simulink model "rlCartPole"  (R2021b)
settings: Solver=VariableStepAuto  StartTime=0.0  StopTime=Tf  RelTol=1e-3
PreLoadFcn:
  | qubeInit
values from neighbouring files (symbols this model uses):
  g = 9.81    [qubeInit.m]
  Jm = 4e-6    (= 4e-06)    [qubeInit.m]
  Klqr = lqr(A,B,Q,R)    [qubeInit.m]
  Lp = 0.129    [qubeInit.m]
  Lr = 0.085    [qubeInit.m]
  maxLimit = 10    [qubeInit.m]
  Mh = 0.0106    [qubeInit.m]
  minLimit = -10    [qubeInit.m]
  Mp = 0.024    [qubeInit.m]
  Mr = 0.095    [qubeInit.m]
  Rh = 0.0111    [qubeInit.m]
  stepFreq = 1    [qubeInit.m]
  stepSize = 0    [qubeInit.m]
  thetaMax = 135    [qubeInit.m]
  Ts = 0.02    [qubeInit.m]
undefined symbols (not defined in the file or in its folder): X, Y, Z
libraries: sm_lib x16, nesl_utility x8, fl_lib x4, rllib x1, ee_lib x1, simulink x1
settings Model: Creator=ndoshi  LastModifiedBy=hooverrj
settings SolverCC: AlgebraicLoopSolver=TrustRegion
settings DataIOCC: TimeSaveName=T  SignalLoggingName=LoggedSigs
settings DebuggingCC: SFMachineParentedDataDiag=warning  ArithmeticOperatorsInVariantConditions=warning
settings SFSimCC: CustomCodeUndefinedFunction=UseInterfaceOnly
settings ExplorerConfigSet: InternalSimMechanicsExplorerSettings="<ExplorerConfiguration><canonicalview>default</canonicalview><AnimationSetting><BasePlaybackSpeed>1.0</BasePlaybackSpeed><PlaybackSpeedFactor>1.0</PlaybackSpeedFactor></AnimationSetting><TilePanel><TileInfo><Tiles Columns=\"1\" Count=\"1\" Rows=\"1\"><Column Weight=\"1\"/><Row Weight=\"1\"/><Tile Height=\"1\" Width=\"1\" X=\"0\" Y=\"0\"/></Tiles></TileInfo><SceneInfo><SceneViewer><BGColor><R>0.60000002384185791</R><G>0.60000002384185791</G><B>0.60000002384185791</B></BGColor><Camera><DoPerspective>on</DoPerspective><Position><X>0.431019807204840122</X><Y>-0.00147907084386321701</Y><Z>0.0248156253974509827</Z></Position><Center><X>0.234686259791210938</X><Y>-0.00147907084386321701</Y><Z>0.0248156253974509827</Z></Center><Up><X>-0</X><Y>0</Y><Z>1</Z></Up><ViewLimDist>1</ViewLimDist><YLim>0.466307658154998583</YLim><XLim>0.677990771454933028</XLim></Camera></SceneViewer></SceneInfo></TilePanel><MechEditorPanel><Cameras><Camera><Id>Camera1</Id><Value><Name>Camera1</Name><NativeCamera><PositionTrackingFeature>Environment.Plant.World_Frame.W</PositionTrackingFeature><CenterTrackingFeature>Environment.Plant.World_Frame.W</CenterTrackingFeature><UpVectorTrackingFeature>Environment.Plant.World_Frame.W</UpVectorTrackingFeature><CenterTrackingOrigin>on</CenterTrackingOrigin><UpVectorTrackingDirection>+X</UpVectorTrackingDirection></NativeCamera></Value></Camera></Cameras><GfxPanelCameraMap><MapElement CameraMLId=\"Camera1\" GfxPanelIndex=\"0\"/></GfxPanelCameraMap><VideoCreator><PlaybackSpeedRatio>1.0</PlaybackSpeedRatio><FrameRate>30</FrameRate><VideoFormat>Motion JPEG AVI</VideoFormat><FrameSize>auto</FrameSize></VideoCreator></MechEditorPanel></ExplorerConfiguration>"

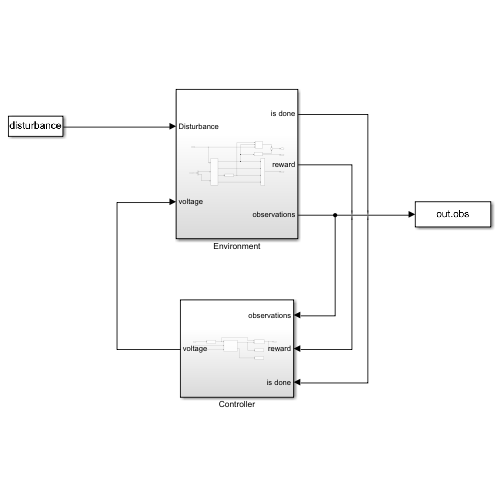
[thumbnail: Simulink's stored preview of the top-level diagram]
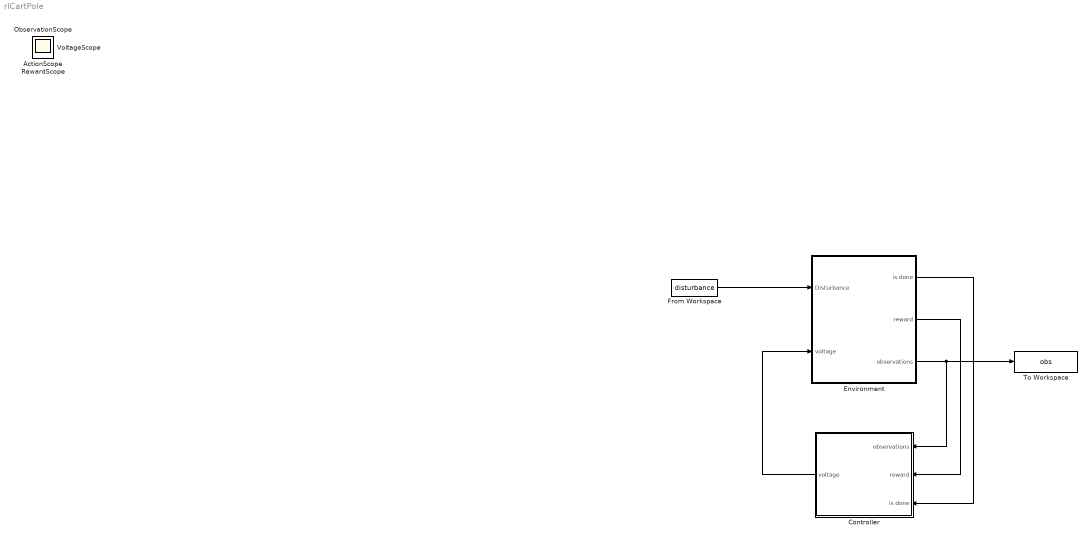
== system rlCartPole ==
  Controller : Subsystem
  Environment : Subsystem
  From Workspace : FromWorkspace  VariableName=disturbance
  To Workspace : ToWorkspace  VariableName=obs  SaveFormat=Timeseries  SampleTime=-1
  ActionScope : Scope
  ObservationScope : Scope
  RewardScope : Scope
  VoltageScope : Scope
  wires:
  Environment/3(observations) -> Controller/1(observations), To Workspace/1
  Environment/2(reward) -> Controller/2(reward)
  Environment/1(is done) -> Controller/3(is done)
  Controller/1(voltage) -> Environment/2(voltage)
  From Workspace/1 -> Environment/1(Disturbance)

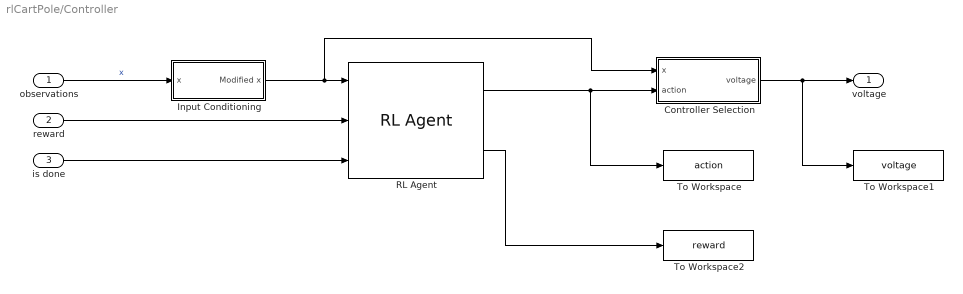
== system rlCartPole/Controller ==
  observations : Inport
  reward : Inport  Port=2
  is done : Inport  Port=3
  Controller Selection : Subsystem  Variant=on
  Input Conditioning : Subsystem
  RL Agent : rllib/RL Agent  Agent=agent  ExternalActionAsInput=off  ProvideCumRwd=on  TreatAsDirectFeedthrough=on
  To Workspace : ToWorkspace  VariableName=action  SaveFormat=Timeseries  SampleTime=-1
  To Workspace1 : ToWorkspace  VariableName=voltage  SaveFormat=Timeseries  SampleTime=-1
  To Workspace2 : ToWorkspace  VariableName=reward  SaveFormat=Timeseries  SampleTime=-1
  voltage : Outport
  wires:
  reward/1 -> RL Agent/2
  is done/1 -> RL Agent/3
  Controller Selection/1(voltage) -> To Workspace1/1, voltage/1
  RL Agent/1 -> To Workspace/1, Controller Selection/2(action)
  Input Conditioning/1(Modified x) -> Controller Selection/1(x), RL Agent/1
  observations/1 -> Input Conditioning/1(x)  "x"
  RL Agent/2 -> To Workspace2/1

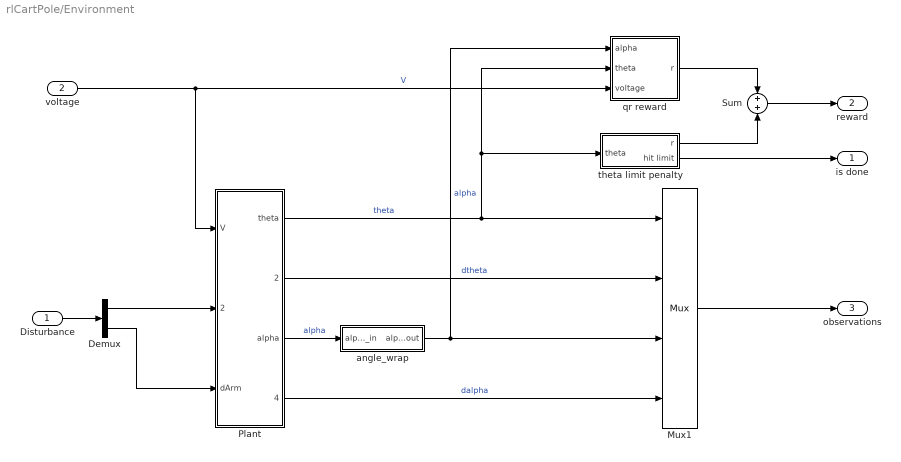
== system rlCartPole/Environment ==
  Disturbance : Inport
  voltage : Inport  Port=2
  Demux : Demux  Outputs=2
  Mux1 : Mux
  Plant : Subsystem
  Sum : Sum
  angle_wrap : Subsystem
  qr reward : Subsystem
  theta limit penalty : Subsystem
  is done : Outport  VectorParamsAs1DForOutWhenUnconnected=off
  reward : Outport  Port=2  VectorParamsAs1DForOutWhenUnconnected=off
  observations : Outport  Port=3  VectorParamsAs1DForOutWhenUnconnected=off
  wires:
  Mux1/1 -> observations/1
  Plant/4(alpha_dot) -> Mux1/4  "dalpha"
  Plant/3(alpha) -> angle_wrap/1(alpha_in)  "alpha"
  Plant/1(theta) -> Mux1/1, qr reward/2(theta), theta limit penalty/1(theta)  "theta"
  angle_wrap/1(alpha_out) -> Mux1/3, qr reward/1(alpha)  "alpha"
  Plant/2(theta_dot) -> Mux1/2  "dtheta"
  Sum/1 -> reward/1
  theta limit penalty/2(hit limit) -> is done/1
  voltage/1 -> Plant/1(V), qr reward/3(voltage)  "V"
  qr reward/1(r) -> Sum/1
  theta limit penalty/1(r) -> Sum/2
  Demux/2 -> Plant/3(dArm)
  Demux/1 -> Plant/2(dPend)
  Disturbance/1 -> Demux/1

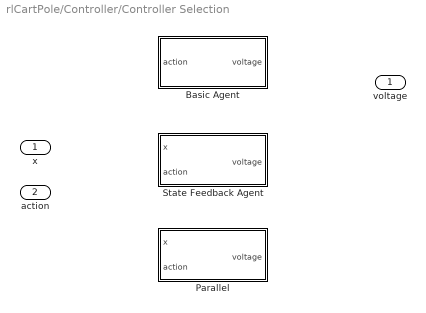
== system rlCartPole/Controller/Controller Selection ==
  x : Inport
  action : Inport  Port=2
  Basic Agent : Subsystem  VariantControl=VSS_CONTROL_BASIC
  Parallel : Subsystem  VariantControl=VSS_CONTROL_FF
  State Feedback Agent : Subsystem  VariantControl=VSS_CONTROL_STATE
  voltage : Outport

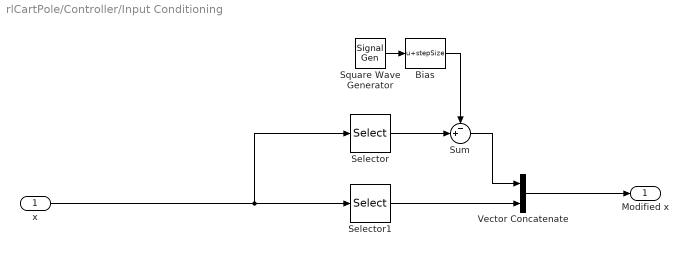
== system rlCartPole/Controller/Input Conditioning ==
  x : Inport
  Bias : Bias  Bias=stepSize
  Selector : Selector  InputPortWidth=4  IndexOptions=Index vector (dialog)  Indices=1  OutputSizes=1
  Selector1 : Selector  InputPortWidth=4  IndexOptions=Index vector (dialog)  Indices=[2 3 4]  OutputSizes=1
  Square Wave Generator : SignalGenerator  WaveForm=square  Amplitude=stepSize  Frequency=stepFreq
  Sum : Sum  Inputs=-+|
  Vector Concatenate : Concatenate
  Modified x : Outport
  wires:
  Vector Concatenate/1 -> Modified x/1
  x/1 -> Selector1/1, Selector/1
  Square Wave Generator/1 -> Bias/1
  Sum/1 -> Vector Concatenate/1
  Selector1/1 -> Vector Concatenate/2
  Selector/1 -> Sum/2
  Bias/1 -> Sum/1

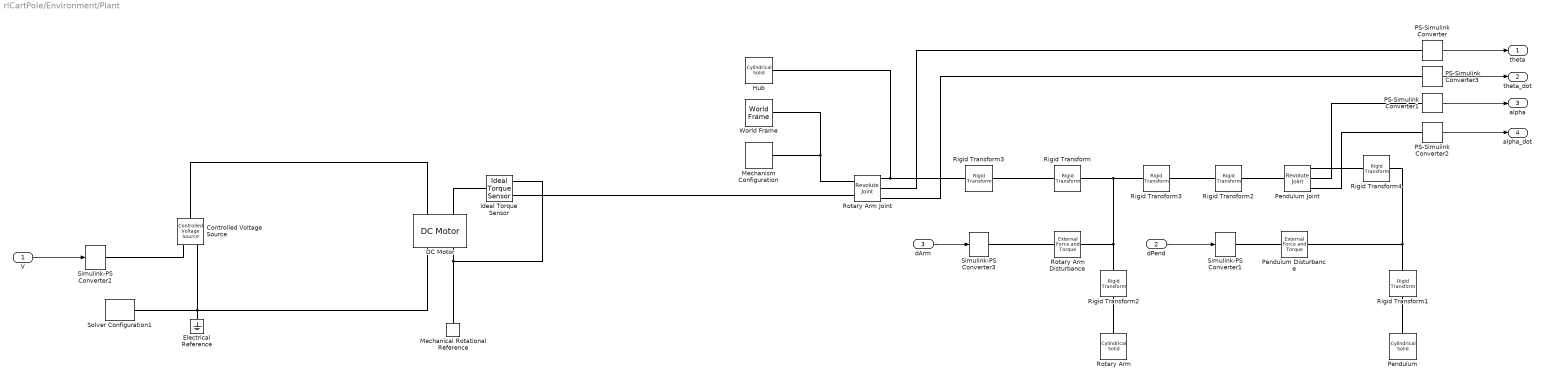
== system rlCartPole/Environment/Plant ==
  V : Inport
  dPend : Inport  Port=2
  dArm : Inport  Port=3
  Controlled Voltage Source : fl_lib/Electrical/Electrical Sources/Controlled Voltage Source
  DC Motor : ee_lib/Electromechanical/Brushed Motors/DC Motor  field_option=ee.enum.field_option.pm  Rf=100 Ohm  Lf=1 H  Laf=0.15 H  If0=0 A  parameterization=1  Ra=Rm Ohm  La=Lm mH  emf_or_torque=1  Kv=Km V/(rad/s)  Ki=6.876e-4 N*m/A  T_stall=0.24e-3 N*m  w_max=19100 rpm  w_rated=15000 rpm  P_rated=0.08 W  V_rated=1.5 V  lam_param=1  i_noload=0 A  V_i_noload=1.5 V  J=Jm kg*m^2  lam=0 N*m/(rad/s)  speed0=0 rpm  enable_fault_armature=simscape.enum.onoff.off  rev_faulted=1 / 3  G_faulted_armature=1e-5 S  fault_trigger_armature=ee.enum.faults.faultTrigger.temporal  t_fault_armature=1 s  max_permissible_current_armature=inf A  t_fail_on_current_armature=1 s  enable_fault_field=simscape.enum.onoff.off  G_faulted_field=1e-5 S  fault_trigger_field=ee.enum.faults.faultTrigger.temporal  t_fault_field=1 s  max_permissible_current_field=inf A  t_fail_on_current_field=1 s  fault_action=simscape.enum.assert.action.none  alpha=3.93e-3 1/K  Tmeas=25 degC  thermal_mass=100 J/K  initial_temperature=25 degC
  Electrical Reference : fl_lib/Electrical/Electrical Elements/Electrical Reference
  Hub : sm_lib/Body Elements/Cylindrical Solid  GraphicAmbientColor=[0.15 0.15 0.15 1.0]  BasedOnType=Mass  CenterOfMass=[0 0 0]  CenterOfMassUnits=m  GraphicDiffuseColor=[0.5 0.5 0.5]  CylinderLength=Rh/2  CylinderLengthUnits=m  CylinderRadius=Rh  CylinderRadiusUnits=m  Density=1000  DensityUnits=kg/m^3  DoExposeReferenceFrame=on  GraphicEmissiveColor=[0.0 0.0 0.0 1.0]  ExportEntireGeometry=off  SerializedFrames=<Frames/>  MarkerShape=Sphere  MarkerSize=10  GraphicType=FromGeometry  InertiaType=CalculateFromGeometry  Mass=Mh  MassUnits=kg  MomentsOfInertia=[1 1 1]  MomentsOfInertiaUnits=kg*m^2  GraphicOpacity=1.0  ProductsOfInertia=[0 0 0]  ProductsOfInertiaUnits=kg*m^2  GraphicShininess=75  GraphicSpecularColor=[0.5 0.5 0.5 1.0]  GraphicVisPropType=SimpleVisualProperties
  Ideal Torque Sensor : fl_lib/Mechanical/Mechanical Sensors/Ideal Torque Sensor
  Mechanical Rotational Reference : fl_lib/Mechanical/Rotational Elements/Mechanical Rotational Reference
  Mechanism Configuration : sm_lib/Utilities/Mechanism Configuration  UniformGravity=Constant  GravityVector=[0 0 -g]  GravityUnits=m/s^2  LinearizationDelta=0.001  JointModeTransitionNonlinearIterations=2
  PS-Simulink Converter{,1..3} (4 alike) : nesl_utility/PS-Simulink Converter  PhysicalDomain=network_engine_domain  SubClassName=ps_output  LeftPortType=input  RightPortType=output  PseudoPeriodic=off  Frequencies=[]  Unit=1  AffineConversion=off
      settings: SourceProductBaseCode=PW,SS
  Pendulum : sm_lib/Body Elements/Cylindrical Solid  GraphicAmbientColor=[0.15 0.15 0.15 1.0]  BasedOnType=Mass  CenterOfMass=[0 0 0]  CenterOfMassUnits=m  GraphicDiffuseColor=[0.8 0.0 0.2]  CylinderLength=Lp  CylinderLengthUnits=m  CylinderRadius=0.005  CylinderRadiusUnits=m  Density=1000  DensityUnits=kg/m^3  DoExposeReferenceFrame=on  GraphicEmissiveColor=[0.0 0.0 0.0 1.0]  ExportEntireGeometry=off  SerializedFrames=<Frames/>  MarkerShape=Sphere  MarkerSize=10  GraphicType=FromGeometry  InertiaType=CalculateFromGeometry  Mass=Mp  MassUnits=kg  MomentsOfInertia=[1 1 1]  MomentsOfInertiaUnits=kg*m^2  GraphicOpacity=1.0  ProductsOfInertia=[0 0 0]  ProductsOfInertiaUnits=kg*m^2  GraphicShininess=75  GraphicSpecularColor=[0.5 0.5 0.5 1.0]  GraphicVisPropType=SimpleVisualProperties
  Pendulum Disturbance : sm_lib/Forces and Torques/External Force and Torque  ForceResolutionFrame=AttachedFrame  EnableForceX=off  EnableForceY=on  EnableForceZ=off  EnableForce=off  TorqueResolutionFrame=AttachedFrame  EnableTorqueX=off  EnableTorqueY=off  EnableTorqueZ=off  EnableTorque=off
  Pendulum Joint : sm_lib/Joints/Revolute Joint  JointMode=Normal  SenseConstraintForce=off  SenseConstraintForceX=off  SenseConstraintForceY=off  SenseConstraintForceZ=off  SenseConstraintTorque=off  SenseConstraintTorqueX=off  SenseConstraintTorqueY=off  SenseConstraintTorqueZ=off  SenseTotalForce=off  SenseTotalForceX=off  SenseTotalForceY=off  SenseTotalForceZ=off  SenseTotalTorque=off  SenseTotalTorqueX=off  SenseTotalTorqueY=off  SenseTotalTorqueZ=off  CompositeWrenchDir=FollowerOnBase  CompositeWrenchFrame=BaseFrame  EquilibriumPosition=0  EquilibriumPositionUnits=deg  SpringStiffness=0  SpringStiffnessUnits=N*m/deg  DampingCoefficient=Dp  DampingCoefficientUnits=N*m/(rad/s)  TorqueActuationMode=NoTorque  MotionActuationMode=ComputedMotion  SensePosition=on  SenseVelocity=on  SenseAcceleration=off  SenseTorqueForce=off  SenseLowerLimitTorqueForce=off  SenseUpperLimitTorqueForce=off  LowerLimitSpecify=off  LowerLimitBound=-90  LowerLimitBoundUnits=deg  LowerLimitStiffness=1e4  LowerLimitStiffnessUnits=N*m/deg  LowerLimitDamping=10  LowerLimitDampingUnits=N*m/(deg/s)  LowerLimitTransitionRegionWidth=0.1  LowerLimitTransitionRegionWidthUnits=deg  UpperLimitSpecify=off  UpperLimitBound=90  UpperLimitBoundUnits=deg  UpperLimitStiffness=1e4  UpperLimitStiffnessUnits=N*m/deg  UpperLimitDamping=10  UpperLimitDampingUnits=N*m/(deg/s)  UpperLimitTransitionRegionWidth=0.1  UpperLimitTransitionRegionWidthUnits=deg  PositionTargetSpecify=on  PositionTargetPriority=High  PositionTargetValue=alpha0  PositionTargetValueUnits=deg  VelocityTargetSpecify=off  VelocityTargetPriority=High  VelocityTargetValue=0  VelocityTargetValueUnits=deg/s
  Rigid Transform : sm_lib/Frames and Transforms/Rigid Transform  TranslationMethod=StandardAxis  TranslationStandardOffset=Lr/2  TranslationLengthUnit=m  TranslationStandardAxis=-X  TranslationCartesianOffset=[0 0 0]  TranslationROffset=0  TranslationROffsetUnits=m  TranslationZOffset=0  TranslationZOffsetUnits=m  TranslationThetaOffset=0  TranslationThetaOffsetUnits=deg  RotationMethod=None  RotationAngleUnits=deg  RotationStandardAxis=+Z  RotationAngle=0.0  RotationArbitraryAxis=[0 0 1]  FollAlignAxisA=+X  BaseAlignAxisA=+Y  FollAlignAxisB=+Y  BaseAlignAxisB=+Z  RotationSequenceAxes=FollowerAxes  RotationSequence=XYX  RotationSequenceAngles=[0 0 0]  RotationSequenceAnglesUnits=deg  RotationMatrix=[1 0 0; 0 1 0; 0 0 1]
  Rigid Transform1 : sm_lib/Frames and Transforms/Rigid Transform  TranslationMethod=None  TranslationStandardOffset=0  TranslationLengthUnit=m  TranslationStandardAxis=+Z  TranslationCartesianOffset=[0 0 0]  TranslationROffset=0  TranslationROffsetUnits=m  TranslationZOffset=0  TranslationZOffsetUnits=m  TranslationThetaOffset=0  TranslationThetaOffsetUnits=deg  RotationMethod=StandardAxis  RotationAngleUnits=deg  RotationStandardAxis=-Y  RotationAngle=90  RotationArbitraryAxis=[0 0 1]  FollAlignAxisA=+X  BaseAlignAxisA=+Y  FollAlignAxisB=+Y  BaseAlignAxisB=+Z  RotationSequenceAxes=FollowerAxes  RotationSequence=XYX  RotationSequenceAngles=[0 0 0]  RotationSequenceAnglesUnits=deg  RotationMatrix=[1 0 0; 0 1 0; 0 0 1]
  Rigid Transform2 : sm_lib/Frames and Transforms/Rigid Transform  TranslationMethod=None  TranslationStandardOffset=0  TranslationLengthUnit=m  TranslationStandardAxis=+Z  TranslationCartesianOffset=[0 0 0]  TranslationROffset=0  TranslationROffsetUnits=m  TranslationZOffset=0  TranslationZOffsetUnits=m  TranslationThetaOffset=0  TranslationThetaOffsetUnits=deg  RotationMethod=StandardAxis  RotationAngleUnits=deg  RotationStandardAxis=-Y  RotationAngle=90  RotationArbitraryAxis=[0 0 1]  FollAlignAxisA=+X  BaseAlignAxisA=+Y  FollAlignAxisB=+Y  BaseAlignAxisB=+Z  RotationSequenceAxes=FollowerAxes  RotationSequence=XYX  RotationSequenceAngles=[0 0 0]  RotationSequenceAnglesUnits=deg  RotationMatrix=[1 0 0; 0 1 0; 0 0 1]
  Rigid Transform3 : sm_lib/Frames and Transforms/Rigid Transform  TranslationMethod=StandardAxis  TranslationStandardOffset=Rh/2  TranslationLengthUnit=m  TranslationStandardAxis=-Z  TranslationCartesianOffset=[0 0 0]  TranslationROffset=0  TranslationROffsetUnits=m  TranslationZOffset=0  TranslationZOffsetUnits=m  TranslationThetaOffset=0  TranslationThetaOffsetUnits=deg  RotationMethod=None  RotationAngleUnits=deg  RotationStandardAxis=+Z  RotationAngle=0.0  RotationArbitraryAxis=[0 0 1]  FollAlignAxisA=+X  BaseAlignAxisA=+Y  FollAlignAxisB=+Y  BaseAlignAxisB=+Z  RotationSequenceAxes=FollowerAxes  RotationSequence=XYX  RotationSequenceAngles=[0 0 0]  RotationSequenceAnglesUnits=deg  RotationMatrix=[1 0 0; 0 1 0; 0 0 1]
  Rigid Transform2 : sm_lib/Frames and Transforms/Rigid Transform  TranslationMethod=StandardAxis  TranslationStandardOffset=Lr/2  TranslationLengthUnit=m  TranslationStandardAxis=+Z  TranslationCartesianOffset=[0 0 0]  TranslationROffset=0  TranslationROffsetUnits=m  TranslationZOffset=0  TranslationZOffsetUnits=m  TranslationThetaOffset=0  TranslationThetaOffsetUnits=deg  RotationMethod=None  RotationAngleUnits=deg  RotationStandardAxis=-X  RotationAngle=90  RotationArbitraryAxis=[0 0 1]  FollAlignAxisA=+X  BaseAlignAxisA=+Y  FollAlignAxisB=+Y  BaseAlignAxisB=+Z  RotationSequenceAxes=FollowerAxes  RotationSequence=XYX  RotationSequenceAngles=[0 0 0]  RotationSequenceAnglesUnits=deg  RotationMatrix=[1 0 0; 0 1 0; 0 0 1]
  Rigid Transform3 : sm_lib/Frames and Transforms/Rigid Transform  TranslationMethod=None  TranslationStandardOffset=0  TranslationLengthUnit=m  TranslationStandardAxis=+Z  TranslationCartesianOffset=[0 0 0]  TranslationROffset=0  TranslationROffsetUnits=m  TranslationZOffset=0  TranslationZOffsetUnits=m  TranslationThetaOffset=0  TranslationThetaOffsetUnits=deg  RotationMethod=StandardAxis  RotationAngleUnits=deg  RotationStandardAxis=+Y  RotationAngle=90  RotationArbitraryAxis=[0 0 1]  FollAlignAxisA=+X  BaseAlignAxisA=+Y  FollAlignAxisB=+Y  BaseAlignAxisB=+Z  RotationSequenceAxes=FollowerAxes  RotationSequence=XYX  RotationSequenceAngles=[0 0 0]  RotationSequenceAnglesUnits=deg  RotationMatrix=[1 0 0; 0 1 0; 0 0 1]
  Rigid Transform4 : sm_lib/Frames and Transforms/Rigid Transform  TranslationMethod=StandardAxis  TranslationStandardOffset=Lp/2  TranslationLengthUnit=m  TranslationStandardAxis=-X  TranslationCartesianOffset=[0 0 0]  TranslationROffset=0  TranslationROffsetUnits=m  TranslationZOffset=0  TranslationZOffsetUnits=m  TranslationThetaOffset=0  TranslationThetaOffsetUnits=deg  RotationMethod=None  RotationAngleUnits=deg  RotationStandardAxis=+X  RotationAngle=90  RotationArbitraryAxis=[0 0 1]  FollAlignAxisA=+X  BaseAlignAxisA=+Y  FollAlignAxisB=+Y  BaseAlignAxisB=+Z  RotationSequenceAxes=FollowerAxes  RotationSequence=XYX  RotationSequenceAngles=[0 0 0]  RotationSequenceAnglesUnits=deg  RotationMatrix=[1 0 0; 0 1 0; 0 0 1]
  Rotary Arm : sm_lib/Body Elements/Cylindrical Solid  GraphicAmbientColor=[0.15 0.15 0.15 1.0]  BasedOnType=Mass  CenterOfMass=[0 0 0]  CenterOfMassUnits=m  GraphicDiffuseColor=[0.5 0.5 0.5]  CylinderLength=Lr  CylinderLengthUnits=m  CylinderRadius=0.003  CylinderRadiusUnits=m  Density=1000  DensityUnits=kg/m^3  DoExposeReferenceFrame=on  GraphicEmissiveColor=[0.0 0.0 0.0 1.0]  ExportEntireGeometry=off  SerializedFrames=<Frames/>  MarkerShape=Sphere  MarkerSize=10  GraphicType=FromGeometry  InertiaType=CalculateFromGeometry  Mass=Mr  MassUnits=kg  MomentsOfInertia=[1 1 1]  MomentsOfInertiaUnits=kg*m^2  GraphicOpacity=1.0  ProductsOfInertia=[0 0 0]  ProductsOfInertiaUnits=kg*m^2  GraphicShininess=75  GraphicSpecularColor=[0.5 0.5 0.5 1.0]  GraphicVisPropType=SimpleVisualProperties
  Rotary Arm Disturbance : sm_lib/Forces and Torques/External Force and Torque  ForceResolutionFrame=AttachedFrame  EnableForceX=off  EnableForceY=on  EnableForceZ=off  EnableForce=off  TorqueResolutionFrame=AttachedFrame  EnableTorqueX=off  EnableTorqueY=off  EnableTorqueZ=off  EnableTorque=off
  Rotary Arm Joint : sm_lib/Joints/Revolute Joint  JointMode=Normal  SenseConstraintForce=off  SenseConstraintForceX=off  SenseConstraintForceY=off  SenseConstraintForceZ=off  SenseConstraintTorque=off  SenseConstraintTorqueX=off  SenseConstraintTorqueY=off  SenseConstraintTorqueZ=off  SenseTotalForce=off  SenseTotalForceX=off  SenseTotalForceY=off  SenseTotalForceZ=off  SenseTotalTorque=off  SenseTotalTorqueX=off  SenseTotalTorqueY=off  SenseTotalTorqueZ=off  CompositeWrenchDir=FollowerOnBase  CompositeWrenchFrame=BaseFrame  EquilibriumPosition=0  EquilibriumPositionUnits=deg  SpringStiffness=0  SpringStiffnessUnits=N*m/deg  DampingCoefficient=Dr  DampingCoefficientUnits=N*m/(rad/s)  TorqueActuationMode=InputTorque  MotionActuationMode=ComputedMotion  SensePosition=on  SenseVelocity=on  SenseAcceleration=off  SenseTorqueForce=off  SenseLowerLimitTorqueForce=off  SenseUpperLimitTorqueForce=off  LowerLimitSpecify=off  LowerLimitBound=-90  LowerLimitBoundUnits=deg  LowerLimitStiffness=1e4  LowerLimitStiffnessUnits=N*m/deg  LowerLimitDamping=10  LowerLimitDampingUnits=N*m/(deg/s)  LowerLimitTransitionRegionWidth=0.1  LowerLimitTransitionRegionWidthUnits=deg  UpperLimitSpecify=off  UpperLimitBound=90  UpperLimitBoundUnits=deg  UpperLimitStiffness=1e4  UpperLimitStiffnessUnits=N*m/deg  UpperLimitDamping=10  UpperLimitDampingUnits=N*m/(deg/s)  UpperLimitTransitionRegionWidth=0.1  UpperLimitTransitionRegionWidthUnits=deg  PositionTargetSpecify=on  PositionTargetPriority=High  PositionTargetValue=theta0  PositionTargetValueUnits=deg  VelocityTargetSpecify=off  VelocityTargetPriority=High  VelocityTargetValue=0  VelocityTargetValueUnits=deg/s
  Simulink-PS Converter1 : nesl_utility/Simulink-PS Converter  PhysicalDomain=network_engine_domain  SubClassName=ps_input  LeftPortType=input  RightPortType=output  PseudoPeriodic=off  Frequencies=[]  NoiseDistribution=none  NoiseParameters=[]  Unit=1  AffineConversion=off  FilteringAndDerivatives=zero  SimscapeFilterOrder=1  InputFilterTimeConstant=0.001  UdotUserProvided=1
      settings: SourceProductBaseCode=PW,SS
  Simulink-PS Converter2 : nesl_utility/Simulink-PS Converter  PhysicalDomain=network_engine_domain  SubClassName=ps_input  LeftPortType=input  RightPortType=output  PseudoPeriodic=off  Frequencies=[]  NoiseDistribution=none  NoiseParameters=[]  Unit=1  AffineConversion=off  FilteringAndDerivatives=zero  SimscapeFilterOrder=1  InputFilterTimeConstant=0.001  UdotUserProvided=1
      settings: SourceProductBaseCode=PW,SS
  Simulink-PS Converter3 : nesl_utility/Simulink-PS Converter  PhysicalDomain=network_engine_domain  SubClassName=ps_input  LeftPortType=input  RightPortType=output  PseudoPeriodic=off  Frequencies=[]  NoiseDistribution=none  NoiseParameters=[]  Unit=1  AffineConversion=off  FilteringAndDerivatives=zero  SimscapeFilterOrder=1  InputFilterTimeConstant=0.001  UdotUserProvided=1
      settings: SourceProductBaseCode=PW,SS
  Solver Configuration1 : nesl_utility/Solver Configuration  PhysicalDomain=network_engine_domain  SubClassName=solver  LeftPortType=input  RightPortType=generic  Tones=[]  Harmonics=[]  SimulateNoise=off  Profile=off  UseLocalSampling=off  EnableSwitchedLinearOptims=on  FrequencyDomain=off  UseCCode=off  RelTol=0.001  AbsTol=1e-06  MinStep=1e-09  ToWorkspace=off  RevertToSquareIcSolve=off  NumHomotopyIterations=100  PhasorMode=off  PhasorModeNumHarmonics=1  DoDC=off  ResidualTolerance=1e-09  UseLocalSolver=off  LocalSolverChoice=NE_BACKWARD_EULER_ADVANCER  LocalSolverSampleTime=0.001  DoFixedCost=off  MaxNonlinIter=3  MaxModeIter=2  ComputeImpulses=off  ImpulseIterations=2  LinearAlgebra=Sparse  EquationFormulation=NE_TIME_EF  DelaysMemoryBudget=1024  AutomaticFiltering=on  FilteringTimeConstant=0.001  PartitionStorageMethod=AS_NEEDED  PartitionMemoryBudget=1024  PartitionMethod=FAST
      settings: SourceProductBaseCode=PW,SS
  World Frame : sm_lib/Frames and Transforms/World Frame
  theta : Outport  VectorParamsAs1DForOutWhenUnconnected=off
  theta_dot : Outport  Port=2  VectorParamsAs1DForOutWhenUnconnected=off
  alpha : Outport  Port=3  VectorParamsAs1DForOutWhenUnconnected=off
  alpha_dot : Outport  Port=4  VectorParamsAs1DForOutWhenUnconnected=off
  wires:
  PS-Simulink Converter1/1 -> alpha/1
  PS-Simulink Converter/1 -> theta/1
  dPend/1 -> Simulink-PS Converter1/1
  PS-Simulink Converter2/1 -> alpha_dot/1
  PS-Simulink Converter3/1 -> theta_dot/1
  V/1 -> Simulink-PS Converter2/1
  dArm/1 -> Simulink-PS Converter3/1
  connections:
  Rotary Arm Disturbance/RConn1 -- Rigid Transform2/RConn1 -- Rigid Transform/LConn1 -- Rigid Transform3/LConn1
  World Frame/RConn1 -- Rotary Arm Joint/LConn1 -- Mechanism Configuration/RConn1
  Pendulum Joint/RConn1 -- Rigid Transform4/LConn1
  Rigid Transform4/RConn1 -- Rigid Transform1/RConn1 -- Pendulum Disturbance/RConn1
  Pendulum Joint/RConn2 -- PS-Simulink Converter1/LConn1
  PS-Simulink Converter/LConn1 -- Rotary Arm Joint/RConn2
  Simulink-PS Converter1/RConn1 -- Pendulum Disturbance/LConn1
  Pendulum Joint/RConn3 -- PS-Simulink Converter2/LConn1
  PS-Simulink Converter3/LConn1 -- Rotary Arm Joint/RConn3
  Rigid Transform2/RConn1 -- Pendulum Joint/LConn1
  Rigid Transform3/RConn1 -- Rigid Transform2/LConn1
  Simulink-PS Converter3/RConn1 -- Rotary Arm Disturbance/LConn1
  Simulink-PS Converter2/RConn1 -- Controlled Voltage Source/RConn1
  Ideal Torque Sensor/LConn1 -- DC Motor/LConn2
  DC Motor/RConn2 -- Ideal Torque Sensor/RConn1 -- Mechanical Rotational Reference/LConn1
  Controlled Voltage Source/LConn1 -- DC Motor/LConn1
  DC Motor/RConn1 -- Electrical Reference/LConn1 -- Solver Configuration1/RConn1 -- Controlled Voltage Source/RConn2
  Rigid Transform1/LConn1 -- Pendulum/RConn1
  Rigid Transform2/LConn1 -- Rotary Arm/RConn1
  Hub/RConn1 -- Rigid Transform3/RConn1 -- Rotary Arm Joint/RConn1
  Rigid Transform/RConn1 -- Rigid Transform3/LConn1
  Rotary Arm Joint/LConn2 -- Ideal Torque Sensor/RConn2

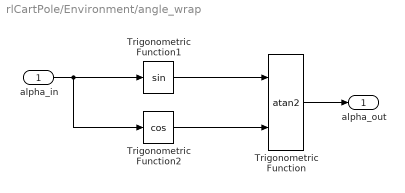
== system rlCartPole/Environment/angle_wrap ==
  alpha_in : Inport
  Trigonometric Function : Trigonometry  Operator=atan2
  Trigonometric Function1 : Trigonometry
  Trigonometric Function2 : Trigonometry  Operator=cos
  alpha_out : Outport  VectorParamsAs1DForOutWhenUnconnected=off
  wires:
  alpha_in/1 -> Trigonometric Function2/1, Trigonometric Function1/1
  Trigonometric Function/1 -> alpha_out/1
  Trigonometric Function1/1 -> Trigonometric Function/1
  Trigonometric Function2/1 -> Trigonometric Function/2

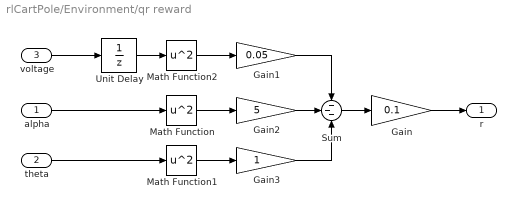
== system rlCartPole/Environment/qr reward ==
  alpha : Inport
  theta : Inport  Port=2
  voltage : Inport  Port=3
  Gain : Gain  Gain=0.1
  Gain1 : Gain  Gain=0.05
  Gain2 : Gain  Gain=5
  Gain3 : Gain
  Math Function : Math  Operator=square  SignedPower=on  SaturateOnIntegerOverflow=on
  Math Function1 : Math  Operator=square  SignedPower=on  SaturateOnIntegerOverflow=on
  Math Function2 : Math  Operator=square  SignedPower=on  SaturateOnIntegerOverflow=on
  Sum : Sum  Inputs=---
  Unit Delay : UnitDelay  SampleTime=Ts  HasFrameUpgradeWarning=on
  r : Outport  VectorParamsAs1DForOutWhenUnconnected=off
  wires:
  Gain2/1 -> Sum/2
  Gain3/1 -> Sum/3
  Math Function2/1 -> Gain1/1
  Math Function1/1 -> Gain3/1
  voltage/1 -> Unit Delay/1
  theta/1 -> Math Function1/1
  Gain1/1 -> Sum/1
  Sum/1 -> Gain/1
  Unit Delay/1 -> Math Function2/1
  Gain/1 -> r/1
  Math Function/1 -> Gain2/1
  alpha/1 -> Math Function/1

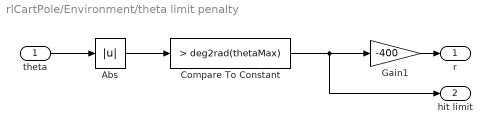
== system rlCartPole/Environment/theta limit penalty ==
  theta : Inport
  Abs : Abs
  Compare To Constant : simulink/Logic and Bit Operations/Compare To Constant  relop=>  const=deg2rad(thetaMax)  OutDataTypeStr=boolean
  Gain1 : Gain  Gain=-400
  r : Outport  VectorParamsAs1DForOutWhenUnconnected=off
  hit limit : Outport  Port=2  VectorParamsAs1DForOutWhenUnconnected=off
  wires:
  Gain1/1 -> r/1
  theta/1 -> Abs/1
  Abs/1 -> Compare To Constant/1
  Compare To Constant/1 -> hit limit/1, Gain1/1

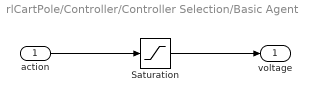
== system rlCartPole/Controller/Controller Selection/Basic Agent ==
  action : Inport
  Saturation : Saturate  UpperLimit=maxLimit  LowerLimit=minLimit
  voltage : Outport
  wires:
  action/1 -> Saturation/1
  Saturation/1 -> voltage/1

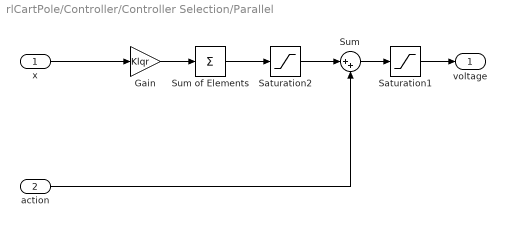
== system rlCartPole/Controller/Controller Selection/Parallel ==
  x : Inport
  action : Inport  Port=2
  Gain : Gain  Gain=Klqr
  Saturation1 : Saturate  UpperLimit=maxLimit  LowerLimit=minLimit
  Saturation2 : Saturate  UpperLimit=maxLimit  LowerLimit=minLimit
  Sum : Sum  Inputs=|++
  Sum of Elements : Sum  Inputs=+
  voltage : Outport
  wires:
  Saturation1/1 -> voltage/1
  x/1 -> Gain/1
  Gain/1 -> Sum of Elements/1
  Sum of Elements/1 -> Saturation2/1
  action/1 -> Sum/2
  Sum/1 -> Saturation1/1
  Saturation2/1 -> Sum/1

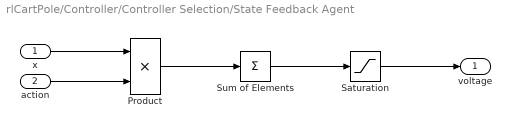
== system rlCartPole/Controller/Controller Selection/State Feedback Agent ==
  x : Inport
  action : Inport  Port=2
  Product : Product
  Saturation : Saturate  UpperLimit=maxLimit  LowerLimit=minLimit
  Sum of Elements : Sum  Inputs=+
  voltage : Outport
  wires:
  Product/1 -> Sum of Elements/1
  Sum of Elements/1 -> Saturation/1
  action/1 -> Product/2
  x/1 -> Product/1
  Saturation/1 -> voltage/1
